simulink model "MECH6313_HW4_pblm3_model"  (R2020b)
settings: Solver=VariableStepAuto  StartTime=0.0  StopTime=10.0  RelTol=1e-3
values from neighbouring files (symbols this model uses):
  a = 1    [runexample.m]
undefined symbols (not defined in the file or in its folder): b, K
libraries: cstblocks x1
settings Model: Creator=Jonas  LastModifiedBy=Jonas

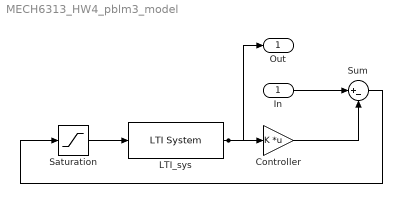
== system MECH6313_HW4_pblm3_model ==
  In : Inport
  Controller : Gain  Gain=K  Multiplication=Matrix(K*u)
  LTI_sys : cstblocks/LTI System  sys=lti_sys  IC=x0
  Saturation : Saturate  UpperLimit=b  LowerLimit=a
  Sum : Sum  Inputs=|+-
  Out : Outport
  wires:
  Saturation/1 -> LTI_sys/1
  Controller/1 -> Sum/2
  Sum/1 -> Saturation/1
  LTI_sys/1 -> Controller/1, Out/1
  In/1 -> Sum/1
